simulink model "ILC_pidQuadsim"  (R2024b)
settings: Solver=VariableStepAuto  StartTime=0.0  StopTime=50  RelTol=1e-3
values from neighbouring files (symbols this model uses):
  tsamp_ILC = 0.10    (= 0.1)    [ILC_setup.m]
undefined symbols (not defined in the file or in its folder): A, B, C, D, pwm, quad
libraries: simulink x2, slctrlobsolete x2, realtime_pacer_lib x2
(part 1 of 2)
settings Model: Creator=elprof  LastModifiedBy=elprof

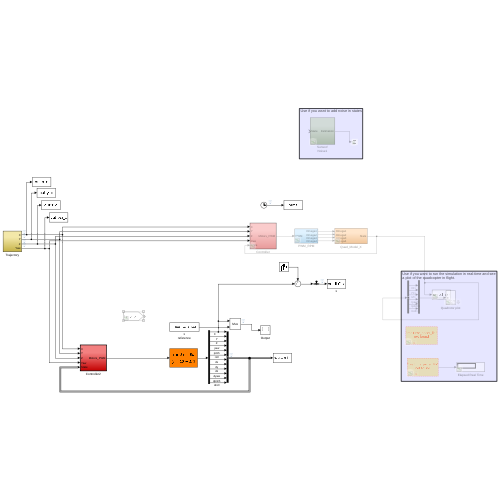
[thumbnail: Simulink's stored preview of the top-level diagram]
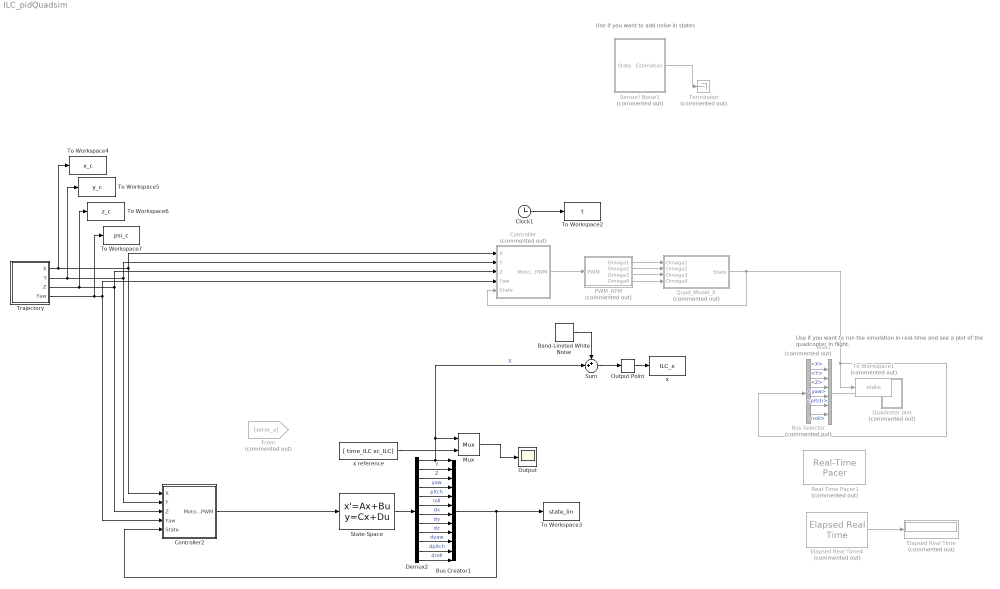
== system ILC_pidQuadsim ==
  note: Use if you want to add noise in states
  note: Use if you want to run the simulation in real-time and see
      | a plot of the quadcopter in flight.
  Band-Limited White Noise : simulink/Sources/Band-Limited White Noise  Cov=[0.0001]*0  Ts=0.1  seed=[23341]
  Bus Creator1 : BusCreator  Inputs=12
  Bus Selector : BusSelector  Commented=on  OutputSignals=X,Y,Z,yaw,pitch,roll
  Clock1 : Clock
  Controller : Subsystem  Commented=on  TreatAsAtomicUnit=on
  Controller2 : Subsystem  TreatAsAtomicUnit=on
  Demux2 : Demux  Outputs=12
  Elapsed Real Time : Display  Commented=on
      settings: Decimation=2
  Elapsed Real Time4 : realtime_pacer_lib/Elapsed Real Time  Commented=on
  From : From  Commented=on  GotoTag=error_x
  Mux : Mux  Inputs=2
  Mux1 : Mux  Commented=on  Inputs=6
  Output : Scope
  Output Point : slctrlobsolete/Output Point
  PWM_RPM : Subsystem  Commented=on
  Quad_Model_X : Subsystem  Commented=on
  Quadrotor plot : Subsystem  Commented=on  AncestorBlock=roblocks/Robot Graphics/Quadrotor plot  mask{quad=quad, xydim=2, zdim=2.3}
      mask prompts: quad "Model"; xydim "xy-axes dimension"; zdim "z-axis dimension"
      mask help: Animate quadrotor.
      mask Help:
      | This block graphically displays a quadrotor (flying robot).
      | 
      | A new figure is created and A graphical model of a quadrotor is animated
      | to a pose specified by the state vector input to the block.
      | 
      | The state vector is [x y z roll pitch yaw] in world coordinates and the
      | angles are in radians.
      | 
      | Notes:
      | - The dimensions of the vehicle workspace are set by parameters
  Real-Time Pacer1 : realtime_pacer_lib/Real-Time Pacer  Commented=on  simTimePerRealTime=1
  Sensor/ Noise1 : Subsystem  Commented=on
  State-Space : StateSpace  A=A  B=B  C=C  D=D  InitialCondition=[0 0 0 0 0 0 0 0 0 0 0 0]'
  Sum : Sum  Inputs=++|  InputSameDT=on  SaturateOnIntegerOverflow=on  OutDataTypeStr=Inherit: Same as first input
  Terminator : Terminator  Commented=on
  To Workspace1 : ToWorkspace  Commented=on  VariableName=state  SampleTime=-1
  To Workspace2 : ToWorkspace  VariableName=t  SampleTime=-1
  To Workspace3 : ToWorkspace  VariableName=state_lin  SampleTime=-1
  To Workspace4 : ToWorkspace  VariableName=x_c  SampleTime=-1
  To Workspace5 : ToWorkspace  VariableName=y_c  SampleTime=-1
  To Workspace6 : ToWorkspace  VariableName=z_c  SampleTime=-1
  To Workspace7 : ToWorkspace  VariableName=psi_c  SampleTime=-1
  Trajectory : Subsystem
  x : ToWorkspace  VariableName=ILC_x  SaveFormat=Structure With Time  SampleTime=-1
  x reference : FromWorkspace  VariableName=[ time_ILC xc_ILC]  SampleTime=tsamp_ILC  ZeroCross=off
  wires:
  Bus Selector/2 -> Mux1/2  "<Y>"
  PWM_RPM/3(Omega3) -> Quad_Model_X/3(Omega3)
  Bus Selector/4 -> Mux1/4  "<yaw>"
  PWM_RPM/2(Omega2) -> Quad_Model_X/2(Omega2)
  Demux2/10 -> Bus Creator1/10  "dyaw"
  PWM_RPM/1(Omega1) -> Quad_Model_X/1(Omega1)
  Demux2/8 -> Bus Creator1/8  "dy"
  Trajectory/2(Y) -> To Workspace5/1, Controller2/2(Y), Controller/2(Y)
  Controller2/1(Motors_PWM) -> State-Space/1
  Bus Selector/1 -> Mux1/1  "<X>"
  Bus Creator1/1 -> To Workspace3/1, Controller2/5(State)
  PWM_RPM/4(Omega4) -> Quad_Model_X/4(Omega4)
  Demux2/5 -> Bus Creator1/5  "pitch"
  Trajectory/3(Z) -> To Workspace6/1, Controller2/3(Z), Controller/3(Z)
  State-Space/1 -> Demux2/1
  Bus Selector/6 -> Mux1/6  "<roll>"
  Demux2/12 -> Bus Creator1/12  "droll"
  Mux1/1 -> Quadrotor plot/1(X)
  Demux2/6 -> Bus Creator1/6  "roll"
  Demux2/3 -> Bus Creator1/3  "Z"
  Demux2/9 -> Bus Creator1/9  "dz"
  Demux2/1 -> Sum/2, Mux/1, Bus Creator1/1  "X"
  Quad_Model_X/1(State) -> Controller/5(State), To Workspace1/1, Bus Selector/1
  Sensor/ Noise1/1(Estimation) -> Terminator/1
  Demux2/11 -> Bus Creator1/11  "dpitch"
  Controller/1(Motors_PWM) -> PWM_RPM/1(PWM)
  Demux2/2 -> Bus Creator1/2  "Y"
  Trajectory/4(Yaw) -> To Workspace7/1, Controller2/4(Yaw), Controller/4(Yaw)
  Demux2/7 -> Bus Creator1/7  "dx"
  Trajectory/1(X) -> To Workspace4/1, Controller2/1(X), Controller/1(X)
  Bus Selector/5 -> Mux1/5  "<pitch>"
  Elapsed Real Time4/1 -> Elapsed Real Time/1
  Clock1/1 -> To Workspace2/1
  Demux2/4 -> Bus Creator1/4  "yaw"
  Bus Selector/3 -> Mux1/3  "<Z>"
  x reference/1 -> Mux/2
  Output Point/1 -> x/1
  Mux/1 -> Output/1
  Sum/1 -> Output Point/1
  Band-Limited White Noise/1 -> Sum/1

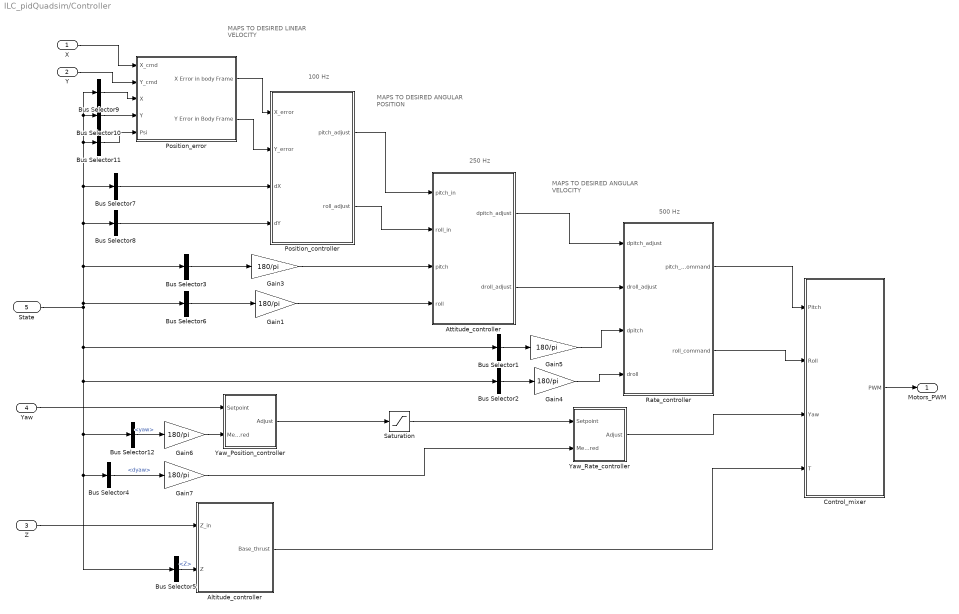
== system ILC_pidQuadsim/Controller ==
  note: 100 Hz
  note: MAPS TO DESIRED
      | ANGULAR VELOCITY
  note: MAPS TO DESIRED
      | ANGULAR POSITION
  note: MAPS TO DESIRED
      | LINEAR VELOCITY
  note: 250 Hz
  note: 500 Hz
  X : Inport
  Y : Inport  Port=2
  Z : Inport  Port=3
  Yaw : Inport  Port=4
  State : Inport  Port=5
  Altitude_controller : Subsystem
  Attitude_controller : Subsystem
  Bus Selector1 : BusSelector  OutputSignals=dpitch  OutputAsBus=on
  Bus Selector10 : BusSelector  OutputSignals=Y  OutputAsBus=on
  Bus Selector11 : BusSelector  OutputSignals=yaw  OutputAsBus=on
  Bus Selector12 : BusSelector  OutputSignals=yaw
  Bus Selector2 : BusSelector  OutputSignals=droll  OutputAsBus=on
  Bus Selector3 : BusSelector  OutputSignals=pitch  OutputAsBus=on
  Bus Selector4 : BusSelector  OutputSignals=dyaw
  Bus Selector5 : BusSelector  OutputSignals=Z
  Bus Selector6 : BusSelector  OutputSignals=roll  OutputAsBus=on
  Bus Selector7 : BusSelector  OutputSignals=dx  OutputAsBus=on
  Bus Selector8 : BusSelector  OutputSignals=dy  OutputAsBus=on
  Bus Selector9 : BusSelector  OutputSignals=X  OutputAsBus=on
  Control_mixer : Subsystem
  Gain{1,3..7} (6 alike) : Gain  Gain=180/pi
  Position_controller : Subsystem
  Position_error : Subsystem
  Rate_controller : Subsystem
  Saturation : Saturate  UpperLimit=200  LowerLimit=-200
  Yaw_Position_controller : Subsystem
  Yaw_Rate_controller : Subsystem
  Motors_PWM : Outport
  wires:
  Control_mixer/1(PWM) -> Motors_PWM/1
  Rate_controller/1(pitch_command) -> Control_mixer/1(Pitch)
  Rate_controller/2(roll_command) -> Control_mixer/2("Roll\t")
  Altitude_controller/1(Base_thrust) -> Control_mixer/4(T)
  Z/1 -> Altitude_controller/1(Z_in)
  Bus Selector5/1 -> Altitude_controller/2(Z)  "<Z>"
  Bus Selector4/1 -> Gain7/1  "<dyaw>"
  State/1 -> Bus Selector9/1, Bus Selector10/1, Bus Selector11/1, Bus Selector7/1, Bus Selector8/1, Bus Selector3/1, Bus Selector6/1, Bus Selector5/1, Bus Selector4/1, Bus Selector12/1, Bus Selector2/1, Bus Selector1/1
  Yaw_Position_controller/1(Adjust) -> Saturation/1
  Yaw_Rate_controller/1(Adjust) -> Control_mixer/3(Yaw)
  Bus Selector6/1 -> Gain1/1
  Attitude_controller/1(dpitch_adjust) -> Rate_controller/1(dpitch_adjust)
  Attitude_controller/2(droll_adjust) -> Rate_controller/2(droll_adjust)
  Bus Selector9/1 -> Position_error/3(X)
  Bus Selector10/1 -> Position_error/4(Y)
  Bus Selector11/1 -> Position_error/5(Psi)
  Position_error/1(X Error in body Frame) -> Position_controller/1(X_error)
  Position_error/2(Y Error in Body Frame) -> Position_controller/2(Y_error)
  Position_controller/1(pitch_adjust) -> Attitude_controller/1(pitch_in)
  Bus Selector3/1 -> Gain3/1
  Gain1/1 -> Attitude_controller/4(roll)
  Gain3/1 -> Attitude_controller/3(pitch)
  Gain4/1 -> Rate_controller/4(droll)
  Gain5/1 -> Rate_controller/3(dpitch)
  Bus Selector1/1 -> Gain5/1
  Bus Selector2/1 -> Gain4/1
  Bus Selector12/1 -> Gain6/1  "<yaw>"
  Gain6/1 -> Yaw_Position_controller/2(Measured)
  Gain7/1 -> Yaw_Rate_controller/2(Measured)
  Position_controller/2(roll_adjust) -> Attitude_controller/2(roll_in)
  X/1 -> Position_error/1(X_cmd)
  Y/1 -> Position_error/2(Y_cmd)
  Bus Selector7/1 -> Position_controller/3(dX)
  Bus Selector8/1 -> Position_controller/4(dY)
  Yaw/1 -> Yaw_Position_controller/1(Setpoint)
  Saturation/1 -> Yaw_Rate_controller/1(Setpoint)

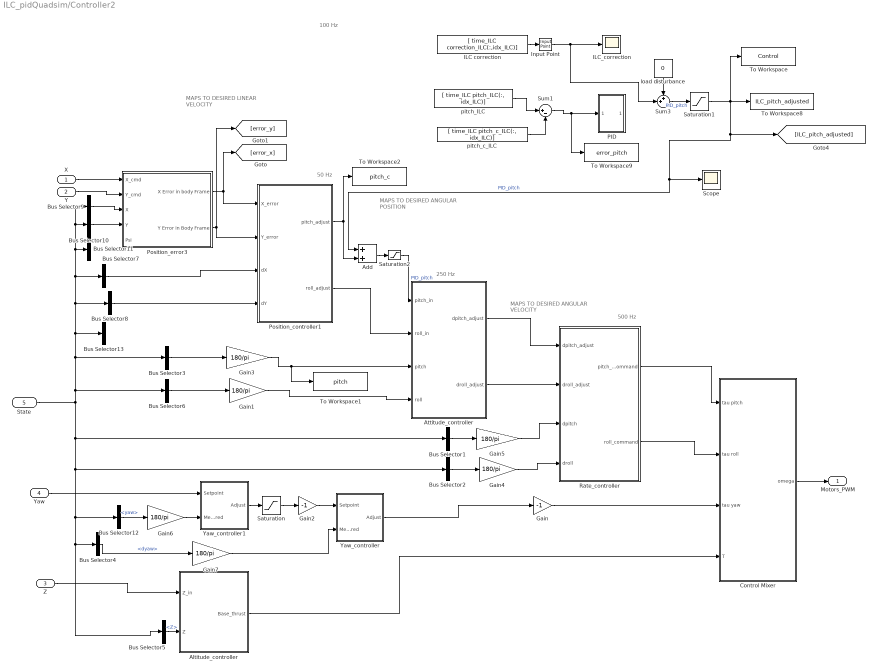
== system ILC_pidQuadsim/Controller2 ==
  note: 500 Hz
  note: 250 Hz
  note: 100 Hz
  note: MAPS TO DESIRED
      | LINEAR VELOCITY
  note: MAPS TO DESIRED
      | ANGULAR POSITION
  note: MAPS TO DESIRED
      | ANGULAR VELOCITY
  note: 50 Hz
  X : Inport
  Y : Inport  Port=2
  Z : Inport  Port=3
  Yaw : Inport  Port=4
  State : Inport  Port=5
  Add : Sum
  Altitude_controller : Subsystem
  Attitude_controller : Subsystem
  Bus Selector1 : BusSelector  OutputSignals=dpitch  OutputAsBus=on
  Bus Selector10 : BusSelector  OutputSignals=Y  OutputAsBus=on
  Bus Selector11 : BusSelector  OutputSignals=yaw  OutputAsBus=on
  Bus Selector12 : BusSelector  OutputSignals=yaw
  Bus Selector13 : BusSelector  OutputSignals=yaw  OutputAsBus=on
  Bus Selector2 : BusSelector  OutputSignals=droll  OutputAsBus=on
  Bus Selector3 : BusSelector  OutputSignals=pitch  OutputAsBus=on
  Bus Selector4 : BusSelector  OutputSignals=dyaw
  Bus Selector5 : BusSelector  OutputSignals=Z
  Bus Selector6 : BusSelector  OutputSignals=roll  OutputAsBus=on
  Bus Selector7 : BusSelector  OutputSignals=dx  OutputAsBus=on
  Bus Selector8 : BusSelector  OutputSignals=dy  OutputAsBus=on
  Bus Selector9 : BusSelector  OutputSignals=X  OutputAsBus=on
  Control Mixer : Subsystem  AncestorBlock=roblocks/Dynamics/Control Mixer 4
      mask help: Quadrotor control mixer
      mask Help:
      | Determine rotor speeds based on desired torques and thrust.
      | 
      | <b>Inputs::</b>
      | 
      | tau pitch (1x1)  desired pitching torque [Nm]
      | tau roll (1x1)   desired rolling torque [Nm]
      | tau yaw (1x1)    desired yawing torque [Nm]
      | T (1x1)          desired thrust [N]
      | 
      | <b>Outputs::</b>
      | 
      | w1 (1x1) angular velocity of rotor 1 [rad]
      | w2 (1x1) angular velocity of rotor 2 [rad]
      | w3 (1x1) angular velocity of rotor 3 [rad]
      | w4 (1x1) angular velocity of rotor 4 [rad]
      | 
      | <b>Notes::</b>
      | 
      | - Assumes the rotor labelling convention of RVC Fig 4.16.
      | - The quadrotor is underactuated and has only 4 inputs.
  Gain : Gain  Gain=-1
  Gain{1,3..7} (6 alike) : Gain  Gain=180/pi
  Gain2 : Gain  Gain=-1
  ILC correction : FromWorkspace  VariableName=[ time_ILC correction_ILC(:,idx_ILC)]  SampleTime=tsamp_ILC  ZeroCross=off
  ILC_correction : Scope
  Input Point : slctrlobsolete/Input Point
  PID : Subsystem  mask{K=0, Ti=100, Td=20}
  Position_controller1 : Subsystem
  Position_error3 : Subsystem
  Rate_controller : Subsystem
  Saturation : Saturate  UpperLimit=200  LowerLimit=-200
  Saturation1 : Saturate  UpperLimit=30  LowerLimit=-30
  Saturation2 : Saturate  UpperLimit=30  LowerLimit=-30
  Scope : Scope
  Sum1 : Sum  Inputs=|+-
  Sum3 : Sum  Inputs=++|  InputSameDT=on  SaturateOnIntegerOverflow=on  OutDataTypeStr=Inherit: Same as first input
  To Workspace : ToWorkspace  VariableName=Control  SaveFormat=Timeseries  SampleTime=-1
  To Workspace1 : ToWorkspace  VariableName=pitch  SaveFormat=Timeseries  SampleTime=-1
  To Workspace2 : ToWorkspace  VariableName=pitch_c  SampleTime=-1
  To Workspace8 : ToWorkspace  VariableName=ILC_pitch_adjusted  SaveFormat=Timeseries  SampleTime=-1
  To Workspace9 : ToWorkspace  VariableName=error_pitch  SaveFormat=Timeseries  SampleTime=-1
  Yaw_controller : Subsystem
  Yaw_controller1 : Subsystem
  load disturbance : Constant  Value=0
  pitch_ILC : FromWorkspace  VariableName=[ time_ILC pitch_ILC(:, idx_ILC)]  SampleTime=tsamp_ILC  ZeroCross=off
  pitch_c_ILC : FromWorkspace  VariableName="[ time_ILC  pitch_c_ILC(:, idx_ILC)]"  SampleTime=tsamp_ILC  ZeroCross=off
  Motors_PWM : Outport
  wires:
  Y/1 -> Position_error3/2(Y_cmd)
  X/1 -> Position_error3/1(X_cmd)
  Gain7/1 -> Yaw_controller/2(Measured)
  Gain6/1 -> Yaw_controller1/2(Measured)
  Bus Selector12/1 -> Gain6/1  "<yaw>"
  Bus Selector2/1 -> Gain4/1
  Bus Selector1/1 -> Gain5/1
  Gain5/1 -> Rate_controller/3(dpitch)
  Gain4/1 -> Rate_controller/4(droll)
  Gain3/1 -> To Workspace1/1, Attitude_controller/3(pitch)
  Gain1/1 -> Attitude_controller/4(roll)
  Bus Selector3/1 -> Gain3/1
  Position_controller1/1(pitch_adjust) -> Add/2, To Workspace2/1
  Bus Selector8/1 -> Position_controller1/4(dY)
  Bus Selector7/1 -> Position_controller1/3(dX)
  Position_error3/2(Y Error in Body Frame) -> Position_controller1/2(Y_error), [error_y]
  Position_error3/1(X Error in body Frame) -> Position_controller1/1(X_error), [error_x]
  Bus Selector10/1 -> Position_error3/4(Y)
  Bus Selector9/1 -> Position_error3/3(X)
  Attitude_controller/2(droll_adjust) -> Rate_controller/2(droll_adjust)
  Attitude_controller/1(dpitch_adjust) -> Rate_controller/1(dpitch_adjust)
  Bus Selector6/1 -> Gain1/1
  Saturation/1 -> Gain2/1
  Gain2/1 -> Yaw_controller/1(Setpoint)
  Yaw/1 -> Yaw_controller1/1(Setpoint)
  Yaw_controller/1(Adjust) -> Gain/1
  Gain/1 -> Control Mixer/3(tau yaw)
  Yaw_controller1/1(Adjust) -> Saturation/1
  State/1 -> Bus Selector1/1, Bus Selector2/1, Bus Selector12/1, Bus Selector4/1, Bus Selector5/1, Bus Selector3/1, Bus Selector7/1, Bus Selector10/1, Bus Selector9/1, Bus Selector11/1, Bus Selector8/1, Bus Selector13/1, Bus Selector6/1
  Bus Selector4/1 -> Gain7/1  "<dyaw>"
  Bus Selector5/1 -> Altitude_controller/2(Z)  "<Z>"
  Z/1 -> Altitude_controller/1(Z_in)
  Altitude_controller/1(Base_thrust) -> Control Mixer/4(T)
  Rate_controller/2(roll_command) -> Control Mixer/2(tau roll)
  Rate_controller/1(pitch_command) -> Control Mixer/1(tau pitch)
  Control Mixer/1(omega) -> Motors_PWM/1
  pitch_c_ILC/1 -> Sum1/2
  ILC correction/1 -> Input Point/1
  Input Point/1 -> Sum3/2, ILC_correction/1
  Sum1/1 -> To Workspace9/1, PID/1(In1)
  pitch_ILC/1 -> Sum1/1
  load disturbance/1 -> Sum3/1
  Sum3/1 -> Saturation1/1  "PID_pitch"
  Add/1 -> Saturation2/1
  Saturation2/1 -> Attitude_controller/1(pitch_in)  "PID_pitch"
  Saturation1/1 -> To Workspace/1, [ILC_pitch_adjusted], Add/1, Scope/1, To Workspace8/1  "PID_pitch"
  Position_controller1/2(roll_adjust) -> Attitude_controller/2(roll_in)

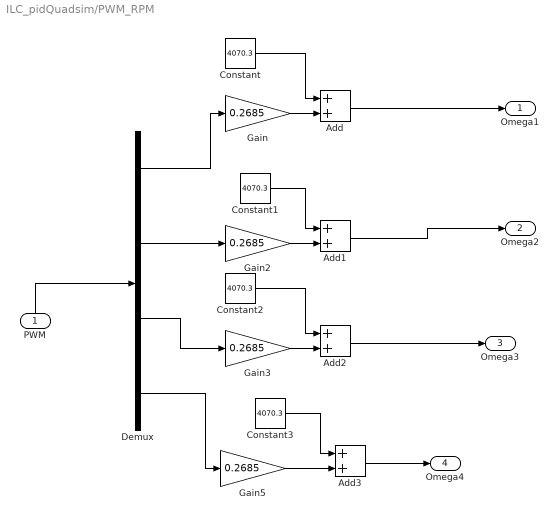
== system ILC_pidQuadsim/PWM_RPM ==
  PWM : Inport
  Add{,1..3} (4 alike) : Sum
  Constant{,1..3} (4 alike) : Constant  Value=4070.3
  Demux : Demux
  Gain{,2..3,5} (4 alike) : Gain  Gain=0.2685
  Omega1 : Outport
  Omega2 : Outport  Port=2
  Omega3 : Outport  Port=3
  Omega4 : Outport  Port=4
  wires:
  Gain/1 -> Add/2
  Demux/1 -> Gain/1
  Demux/4 -> Gain5/1
  Gain5/1 -> Add3/2
  Constant3/1 -> Add3/1
  Add3/1 -> Omega4/1
  Constant1/1 -> Add1/1
  Gain2/1 -> Add1/2
  Demux/2 -> Gain2/1
  Add1/1 -> Omega2/1
  PWM/1 -> Demux/1
  Add/1 -> Omega1/1
  Add2/1 -> Omega3/1
  Demux/3 -> Gain3/1
  Constant2/1 -> Add2/1
  Gain3/1 -> Add2/2
  Constant/1 -> Add/1

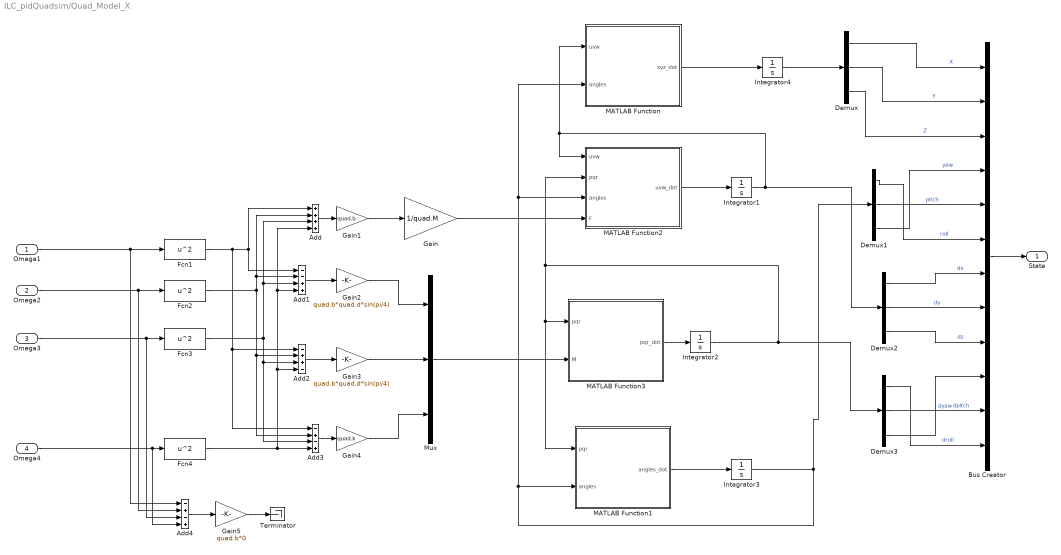
== system ILC_pidQuadsim/Quad_Model_X ==
  Omega1 : Inport
  Omega2 : Inport  Port=2
  Omega3 : Inport  Port=3
  Omega4 : Inport  Port=4
  Add : Sum  Inputs=++++
  Add1 : Sum  Inputs=--++
  Add2 : Sum  Inputs=-++-
  Add3 : Sum  Inputs=-+-+
  Add4 : Sum  Inputs=-+-+
  Bus Creator : BusCreator  Inputs=12
  Demux{,1..3} (4 alike) : Demux  Outputs=3
  Fcn{1..4} (4 alike) : Fcn  Expr=u^2
  Gain : Gain  Gain=1/quad.M
  Gain1 : Gain  Gain=quad.b
  Gain2 : Gain  Gain=quad.b*quad.d*sin(pi/4)
  Gain3 : Gain  Gain=quad.b*quad.d*sin(pi/4)
  Gain4 : Gain  Gain=quad.k
  Gain5 : Gain  Gain=quad.b*0
  Integrator1 : Integrator
  Integrator2 : Integrator
  Integrator3 : Integrator
  Integrator4 : Integrator  InitialCondition=[0;0;0]
  MATLAB Function : MATLAB Function  TreatAsAtomicUnit=on
  MATLAB Function1 : MATLAB Function  TreatAsAtomicUnit=on
  MATLAB Function2 : MATLAB Function  TreatAsAtomicUnit=on
  MATLAB Function3 : MATLAB Function  TreatAsAtomicUnit=on
  Mux : Mux  Inputs=3
  Terminator : Terminator
  State : Outport
  wires:
  Gain1/1 -> Gain/1
  Fcn4/1 -> Add/4, Add1/4, Add2/4, Add3/4
  Fcn3/1 -> Add1/3, Add/3, Add2/3, Add3/3
  Fcn2/1 -> Add2/2, Add3/2, Add1/2, Add/2
  Fcn1/1 -> Add/1, Add1/1, Add2/1, Add3/1
  Bus Creator/1 -> State/1
  Add1/1 -> Gain2/1
  Add/1 -> Gain1/1
  Omega2/1 -> Add4/2, Fcn2/1
  Omega1/1 -> Fcn1/1, Add4/1
  Add2/1 -> Gain3/1
  Gain2/1 -> Mux/1
  Gain4/1 -> Mux/3
  Omega3/1 -> Add4/3, Fcn3/1
  Omega4/1 -> Fcn4/1, Add4/4
  Add4/1 -> Gain5/1
  Add3/1 -> Gain4/1
  Gain3/1 -> Mux/2
  Gain/1 -> MATLAB Function2/4(F)
  Mux/1 -> MATLAB Function3/2(M)
  MATLAB Function/1(xyz_dot) -> Integrator4/1
  MATLAB Function2/1(uvw_dot) -> Integrator1/1
  MATLAB Function3/1(pqr_dot) -> Integrator2/1
  MATLAB Function1/1(angles_dot) -> Integrator3/1
  Integrator3/1 -> Demux1/1, MATLAB Function/2(angles), MATLAB Function2/3(angles), MATLAB Function1/2(angles)
  Integrator1/1 -> Demux2/1, MATLAB Function/1(uvw), MATLAB Function2/1(uvw)
  Integrator2/1 -> Demux3/1, MATLAB Function2/2(pqr), MATLAB Function1/1(pqr), MATLAB Function3/1(pqr)
  Integrator4/1 -> Demux/1
  Demux/1 -> Bus Creator/1  "X"
  Demux/2 -> Bus Creator/2  "Y"
  Demux/3 -> Bus Creator/3  "Z"
  Demux1/3 -> Bus Creator/4  "yaw"
  Demux1/1 -> Bus Creator/6  "roll"
  Demux2/1 -> Bus Creator/7  "dx"
  Demux2/2 -> Bus Creator/8  "dy"
  Demux2/3 -> Bus Creator/9  "dz"
  Demux3/3 -> Bus Creator/10  "dyaw"
  Demux3/2 -> Bus Creator/11  "dpitch"
  Demux3/1 -> Bus Creator/12  "droll"
  Gain5/1 -> Terminator/1
  Demux1/2 -> Bus Creator/5  "pitch"

== system ILC_pidQuadsim/Quadrotor plot ==
  X : Inport
  Plotter : S-Function  FunctionName=quadrotor_plot  Parameters=[xydim, zdim], 1, 1,quad  SFunctionDeploymentMode=off  EnableBusSupport=off
  wires:
  X/1 -> Plotter/1

== system ILC_pidQuadsim/Sensor// Noise1 ==
  note: state
  State : Inport
  Bus Creator : BusCreator  Inputs=2
  Bus Creator1 : BusCreator  Inputs=3
  Bus Selector7 : BusSelector  OutputSignals=X,Y,Z
  Bus Selector8 : BusSelector  OutputSignals=yaw,pitch,roll,dx,dy,dz,dyaw,dpitch,droll  OutputAsBus=on
  Error_X1 : Gain  Gain=0.04
  Error_Y : Gain  Gain=0.04
  Error_Z : Gain  Gain=0.04
  Random Number1 : RandomNumber  SampleTime=0.1
  Random Number2 : RandomNumber  SampleTime=0.1
  Random Number3 : RandomNumber  SampleTime=0.1
  Sum5 : Sum  Inputs=++|
  Sum6 : Sum  Inputs=++|
  Sum7 : Sum  Inputs=++|
  Estimation : Outport
  wires:
  State/1 -> Bus Selector8/1, Bus Selector7/1
  Error_X1/1 -> Sum5/1
  Bus Selector8/1 -> Bus Creator/2
  Random Number3/1 -> Error_X1/1
  Bus Creator/1 -> Estimation/1
  Bus Selector7/1 -> Sum5/2  "<X>"
  Bus Selector7/2 -> Sum6/2  "<Y>"
  Bus Selector7/3 -> Sum7/2  "<Z>"
  Sum5/1 -> Bus Creator1/1  "X'"
  Sum6/1 -> Bus Creator1/2  "Y'"
  Sum7/1 -> Bus Creator1/3  "Z'"
  Bus Creator1/1 -> Bus Creator/1
  Random Number1/1 -> Error_Y/1
  Error_Y/1 -> Sum6/1
  Random Number2/1 -> Error_Z/1
  Error_Z/1 -> Sum7/1

== system ILC_pidQuadsim/Trajectory ==
  Constant3 : Constant
  Ramp2 : simulink/Sources/Ramp  slope=60  start=0  InitialOutput=0
  x* : Sin  Amplitude=0.8  Frequency=2*pi*0.085  Phase=0-0.1  SampleTime=0
  y*1 : Sin  Amplitude=0.8  Frequency=2*pi*0.085  Phase=pi/2-0.1  SampleTime=0
  X : Outport
  Y : Outport  Port=2
  Z : Outport  Port=3
  Yaw : Outport  Port=4
  wires:
  Ramp2/1 -> Yaw/1
  y*1/1 -> Y/1
  x*/1 -> X/1
  Constant3/1 -> Z/1

== system ILC_pidQuadsim/Controller/Altitude_controller ==
  Z_in : Inport
  Z : Inport  Port=2
  "Min_thrust " : Constant  Value=pwm  SampleTime=0
  PID_Altitude : Subsystem
  Saturation : Saturate  UpperLimit=60000  LowerLimit=-20000
  Saturation1 : Saturate  UpperLimit=15000  LowerLimit=-20000
  Sum3 : Sum  Inputs=|++
  Base_thrust : Outport
  wires:
  Saturation/1 -> Base_thrust/1
  "Min_thrust "/1 -> Sum3/2
  Sum3/1 -> Saturation/1
  Z/1 -> PID_Altitude/2(Measured)
  Z_in/1 -> PID_Altitude/1(Setpoint)
  Saturation1/1 -> Sum3/1
  PID_Altitude/1(Adjust) -> Saturation1/1

== system ILC_pidQuadsim/Controller/Attitude_controller ==
  pitch_in : Inport
  roll_in : Inport  Port=2
  pitch : Inport  Port=3
  roll : Inport  Port=4
  PID_Pitch1 : Subsystem
  PID_Pitch3 : Subsystem
  PID_Pitch_Rate2 : Subsystem
  PID_Roll_Rate1 : Subsystem
  dpitch_adjust : Outport
  droll_adjust : Outport  Port=2
  wires:
  roll_in/1 -> PID_Roll_Rate1/1(Setpoint)
  roll/1 -> PID_Roll_Rate1/2(Measured)
  PID_Roll_Rate1/1(Adjust) -> droll_adjust/1
  pitch_in/1 -> PID_Pitch_Rate2/1(Setpoint)
  pitch/1 -> PID_Pitch_Rate2/2(Measured)
  PID_Pitch_Rate2/1(Adjust) -> dpitch_adjust/1

== system ILC_pidQuadsim/Controller/Control_mixer ==
  Pitch : Inport
  "Roll\t" : Inport  Port=2
  Yaw : Inport  Port=3
  T : Inport  Port=4
  Configuration_+ : Subsystem
  Configuration_X1 : Subsystem
  Mode_Selector : Constant  Value=2
  Multiport Switch : MultiPortSwitch  Inputs=2  SaturateOnIntegerOverflow=off  InputSameDT=off
  Mux : Mux
  Mux1 : Mux
  PWM : Outport
  wires:
  Pitch/1 -> Configuration_X1/1(Pitch), Configuration_+/1(Pitch)
  Configuration_X1/3(W3) -> Mux1/3
  Mux1/1 -> Multiport Switch/3
  Mux/1 -> Multiport Switch/2
  Configuration_X1/4(W4) -> Mux1/4
  T/1 -> Configuration_X1/4(Tau), Configuration_+/4(Tau)
  Multiport Switch/1 -> PWM/1
  Yaw/1 -> Configuration_X1/3(Yaw), Configuration_+/3(Yaw)
  "Roll\t"/1 -> Configuration_X1/2(Roll), Configuration_+/2(Roll)
  Mode_Selector/1 -> Multiport Switch/1
  Configuration_+/2(W2) -> Mux/2
  Configuration_+/1(W1) -> Mux/1
  Configuration_X1/2(W2) -> Mux1/2
  Configuration_X1/1(W1) -> Mux1/1
  Configuration_+/3(W3) -> Mux/3
  Configuration_+/4(W4) -> Mux/4

== system ILC_pidQuadsim/Controller/Position_controller ==
  X_error : Inport
  Y_error : Inport  Port=2
  dX : Inport  Port=3
  dY : Inport  Port=4
  PID_Roll_Rate2 : Subsystem
  PID_Roll_Rate3 : Subsystem
  PID_X2 : Subsystem
  PID_Y2 : Subsystem
  Saturation : Saturate  UpperLimit=30  LowerLimit=-30
  Saturation1 : Saturate  UpperLimit=30  LowerLimit=-30
  Scope1 : Scope
  Scope2 : Scope
  pitch_adjust : Outport
  roll_adjust : Outport  Port=2
  wires:
  Saturation1/1 -> roll_adjust/1
  PID_Roll_Rate3/1(Adjust) -> Saturation1/1
  Saturation/1 -> pitch_adjust/1, Scope1/1
  PID_Roll_Rate2/1(Adjust) -> Saturation/1, Scope2/1
  dX/1 -> PID_Roll_Rate2/2(Measured)
  X_error/1 -> PID_Roll_Rate2/1(Setpoint)
  dY/1 -> PID_Roll_Rate3/2(Measured)
  Y_error/1 -> PID_Roll_Rate3/1(Setpoint)

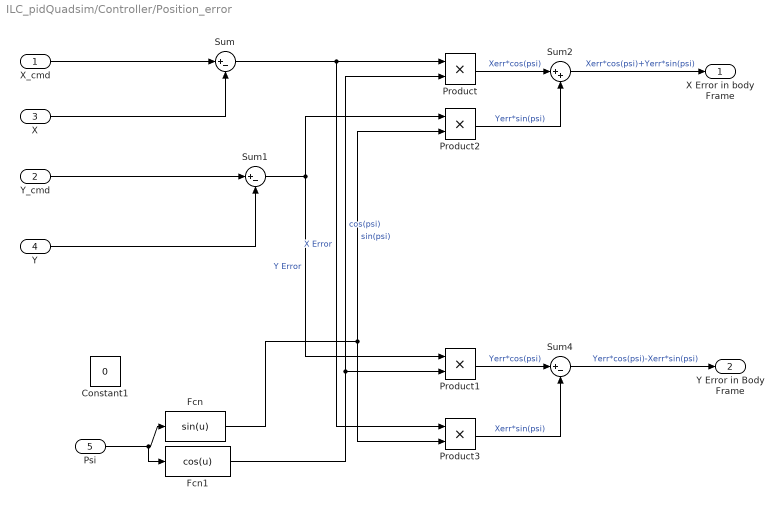
== system ILC_pidQuadsim/Controller/Position_error ==
  X_cmd : Inport
  Y_cmd : Inport  Port=2
  X : Inport  Port=3
  Y : Inport  Port=4
  Psi : Inport  Port=5
  Constant1 : Constant  Value=0
  Fcn : Fcn  Expr=sin(u)
  Fcn1 : Fcn  Expr=cos(u)
  Product{,1..3} (4 alike) : Product
  Sum : Sum  Inputs=|+-
  Sum1 : Sum  Inputs=|+-
  Sum2 : Sum  Inputs=|++
  Sum4 : Sum  Inputs=|+-
  X Error in body Frame : Outport
  Y Error in Body Frame : Outport  Port=2
  wires:
  Sum4/1 -> Y Error in Body Frame/1  "Yerr*cos(psi)-Xerr*sin(psi)"
  Product3/1 -> Sum4/2  "Xerr*sin(psi)"
  Sum1/1 -> Product2/1, Product1/1  "Y Error"
  Fcn/1 -> Product3/2, Product2/2  "sin(psi)"
  Sum2/1 -> X Error in body Frame/1  "Xerr*cos(psi)+Yerr*sin(psi)"
  Y_cmd/1 -> Sum1/1
  X_cmd/1 -> Sum/1
  X/1 -> Sum/2
  Y/1 -> Sum1/2
  Sum/1 -> Product3/1, Product/1  "X Error"
  Fcn1/1 -> Product/2, Product1/2  "cos(psi)"
  Product/1 -> Sum2/1  "Xerr*cos(psi)"
  Product2/1 -> Sum2/2  "Yerr*sin(psi)"
  Product1/1 -> Sum4/1  "Yerr*cos(psi)"
  Psi/1 -> Fcn1/1, Fcn/1

== system ILC_pidQuadsim/Controller/Rate_controller ==
  dpitch_adjust : Inport
  droll_adjust : Inport  Port=2
  dpitch : Inport  Port=3
  droll : Inport  Port=4
  PID_Pitch_Rate1 : Subsystem
  PID_Pitch_Rate3 : Subsystem
  PID_Roll_Rate1 : Subsystem
  PID_Roll_Rate3 : Subsystem
  pitch_command : Outport
  roll_command : Outport  Port=2
  wires:
  dpitch_adjust/1 -> PID_Roll_Rate3/1(Setpoint)
  PID_Roll_Rate3/1(Adjust) -> pitch_command/1
  droll_adjust/1 -> PID_Roll_Rate1/1(Setpoint)
  droll/1 -> PID_Roll_Rate1/2(Measured)
  PID_Roll_Rate1/1(Adjust) -> roll_command/1
  dpitch/1 -> PID_Roll_Rate3/2(Measured)

== system ILC_pidQuadsim/Controller/Yaw_Position_controller ==
  Setpoint : Inport
  Measured : Inport  Port=2
  1/dt : Gain  Gain=1/100  OutMin=[-200]  OutMax=[200]
  Kd : Gain  Gain=0  OutMin=[-200]  OutMax=[200]
  Ki : Gain  Gain=0  OutMin=[-200]  OutMax=[200]
  Kp : Gain  Gain=3  OutMin=[-200]  OutMax=[200]
  Memory : Memory
  Memory1 : Memory
  Saturation : Saturate  UpperLimit=166.7  LowerLimit=-166.7
  Sum1 : Sum  Inputs=|++
  Sum2 : Sum  Inputs=|+-
  Sum5 : Sum  Inputs=+++
  Sum6 : Sum  Inputs=+-|
  dt : Gain  Gain=1/100  OutMin=[-200]  OutMax=[200]
  Adjust : Outport
  wires:
  Measured/1 -> Sum6/2  "measured"
  Setpoint/1 -> Sum6/1  "pid_desired"
  Memory/1 -> Sum2/2  "pid_prevError"
  Ki/1 -> Sum5/2
  Sum5/1 -> Adjust/1
  Kp/1 -> Sum5/1
  Kd/1 -> Sum5/3
  dt/1 -> Sum1/1
  Sum2/1 -> 1/dt/1
  1/dt/1 -> Kd/1
  Sum6/1 -> Sum2/1, Memory/1, dt/1, Kp/1  "pid_error"
  Sum1/1 -> Memory1/1, Saturation/1  "pid_integ"
  Memory1/1 -> Sum1/2
  Saturation/1 -> Ki/1

== system ILC_pidQuadsim/Controller/Yaw_Rate_controller ==
  Setpoint : Inport
  Measured : Inport  Port=2
  1/dt : Gain  Gain=1/500  OutMin=[-200]  OutMax=[200]
  Kd : Gain  Gain=0  OutMin=[-200]  OutMax=[200]
  Ki : Gain  Gain=16.7  OutMin=[-200]  OutMax=[200]
  Kp : Gain  Gain=70  OutMin=[-200]  OutMax=[200]
  Memory : Memory
  Memory1 : Memory
  Saturation : Saturate  UpperLimit=166.7  LowerLimit=-166.7
  Sum1 : Sum  Inputs=|++
  Sum2 : Sum  Inputs=|+-
  Sum5 : Sum  Inputs=+++
  Sum6 : Sum  Inputs=+-|
  dt : Gain  Gain=1/500  OutMin=[-200]  OutMax=[200]
  Adjust : Outport
  wires:
  Measured/1 -> Sum6/2  "measured"
  Setpoint/1 -> Sum6/1  "pid_desired"
  Memory/1 -> Sum2/2  "pid_prevError"
  Ki/1 -> Sum5/2
  Sum5/1 -> Adjust/1
  Kp/1 -> Sum5/1
  Kd/1 -> Sum5/3
  dt/1 -> Sum1/1
  Sum2/1 -> 1/dt/1
  1/dt/1 -> Kd/1
  Sum6/1 -> Sum2/1, Memory/1, dt/1, Kp/1  "pid_error"
  Sum1/1 -> Memory1/1, Saturation/1  "pid_integ"
  Memory1/1 -> Sum1/2
  Saturation/1 -> Ki/1

== system ILC_pidQuadsim/Controller2/Altitude_controller ==
  Z_in : Inport
  Z : Inport  Port=2
  "Min_thrust " : Constant  Value=0  SampleTime=0
  PID_Altitude : Subsystem
  Saturation : Saturate  UpperLimit=60000  LowerLimit=-20000
  Saturation1 : Saturate  UpperLimit=15000  LowerLimit=-20000
  Sum3 : Sum  Inputs=|++
  Base_thrust : Outport
  wires:
  PID_Altitude/1(Adjust) -> Saturation1/1
  Saturation1/1 -> Sum3/1
  Z_in/1 -> PID_Altitude/1(Setpoint)
  Z/1 -> PID_Altitude/2(Measured)
  Sum3/1 -> Saturation/1
  "Min_thrust "/1 -> Sum3/2
  Saturation/1 -> Base_thrust/1

== system ILC_pidQuadsim/Controller2/Attitude_controller ==
  pitch_in : Inport
  roll_in : Inport  Port=2
  pitch : Inport  Port=3
  roll : Inport  Port=4
  PID_Pitch1 : Subsystem
  PID_Pitch3 : Subsystem
  PID_Roll_Rate1 : Subsystem
  PID_Roll_Rate2 : Subsystem
  dpitch_adjust : Outport
  droll_adjust : Outport  Port=2
  wires:
  PID_Roll_Rate2/1(Adjust) -> dpitch_adjust/1
  pitch/1 -> PID_Roll_Rate2/2(Measured)
  pitch_in/1 -> PID_Roll_Rate2/1(Setpoint)
  PID_Roll_Rate1/1(Adjust) -> droll_adjust/1
  roll/1 -> PID_Roll_Rate1/2(Measured)
  roll_in/1 -> PID_Roll_Rate1/1(Setpoint)

== system ILC_pidQuadsim/Controller2/Control Mixer ==
  tau pitch : Inport
  tau roll : Inport  Port=2
  tau yaw : Inport  Port=3
  T : Inport  Port=4
  Configuration_+ : Subsystem
  Configuration_X1 : Subsystem
  Configuration_X2 : Subsystem
  Mode_Selector : Constant  Value=2
  Multiport Switch : MultiPortSwitch  Inputs=2  SaturateOnIntegerOverflow=off  InputSameDT=off
  Mux : Mux
  Mux1 : Mux
  omega : Outport
  wires:
  Mux/1 -> Multiport Switch/2
  Multiport Switch/1 -> omega/1
  Mode_Selector/1 -> Multiport Switch/1
  T/1 -> Configuration_+/4(Tau), Configuration_X1/4(Tau)
  tau yaw/1 -> Configuration_+/3(Yaw), Configuration_X1/3(Yaw)
  tau roll/1 -> Configuration_+/2(Roll), Configuration_X1/2(Roll)
  tau pitch/1 -> Configuration_+/1(Pitch), Configuration_X1/1(Pitch)
  Mux1/1 -> Multiport Switch/3
  Configuration_X1/4(W4) -> Mux1/4
  Configuration_X1/3(W3) -> Mux1/3
  Configuration_X1/2(W2) -> Mux1/2
  Configuration_X1/1(W1) -> Mux1/1
  Configuration_+/4(W4) -> Mux/4
  Configuration_+/3(W3) -> Mux/3
  Configuration_+/2(W2) -> Mux/2
  Configuration_+/1(W1) -> Mux/1

== system ILC_pidQuadsim/Controller2/PID ==
  In1 : Inport
  1/Ti : Gain  Gain=1/Ti  SaturateOnIntegerOverflow=on  OutDataTypeStr=Inherit: Same as input  ParamDataTypeStr=Inherit: Same as input
  Integrator : Integrator
  K : Gain  Gain=K  SaturateOnIntegerOverflow=on  OutDataTypeStr=Inherit: Same as input  ParamDataTypeStr=Inherit: Same as input
  Sum1 : Sum  Inputs=+++  InputSameDT=on  SaturateOnIntegerOverflow=on  OutDataTypeStr=Inherit: Same as first input
  Transfer Fcn1 : TransferFcn  Numerator=[Td 0]  Denominator=[Td/10 1]
  Out1 : Outport
  wires:
  In1/1 -> K/1
  K/1 -> 1/Ti/1, Transfer Fcn1/1, Sum1/1
  1/Ti/1 -> Integrator/1
  Sum1/1 -> Out1/1
  Integrator/1 -> Sum1/2
  Transfer Fcn1/1 -> Sum1/3

== system ILC_pidQuadsim/Controller2/Position_controller1 ==
  X_error : Inport
  Y_error : Inport  Port=2
  dX : Inport  Port=3
  dY : Inport  Port=4
  PID_Roll_Rate2 : Subsystem
  PID_Roll_Rate3 : Subsystem
  PID_X2 : Subsystem
  PID_Y2 : Subsystem
  Saturation : Saturate  UpperLimit=30  LowerLimit=-30
  Saturation1 : Saturate  UpperLimit=30  LowerLimit=-30
  Scope1 : Scope
  Scope2 : Scope
  pitch_adjust : Outport
  roll_adjust : Outport  Port=2
  wires:
  PID_Roll_Rate3/1(Adjust) -> Saturation1/1
  Y_error/1 -> PID_Roll_Rate3/1(Setpoint)
  Saturation1/1 -> roll_adjust/1
  dY/1 -> PID_Roll_Rate3/2(Measured)
  dX/1 -> PID_Roll_Rate2/2(Measured)
  Saturation/1 -> Scope1/1, pitch_adjust/1
  X_error/1 -> PID_Roll_Rate2/1(Setpoint)
  PID_Roll_Rate2/1(Adjust) -> Scope2/1, Saturation/1

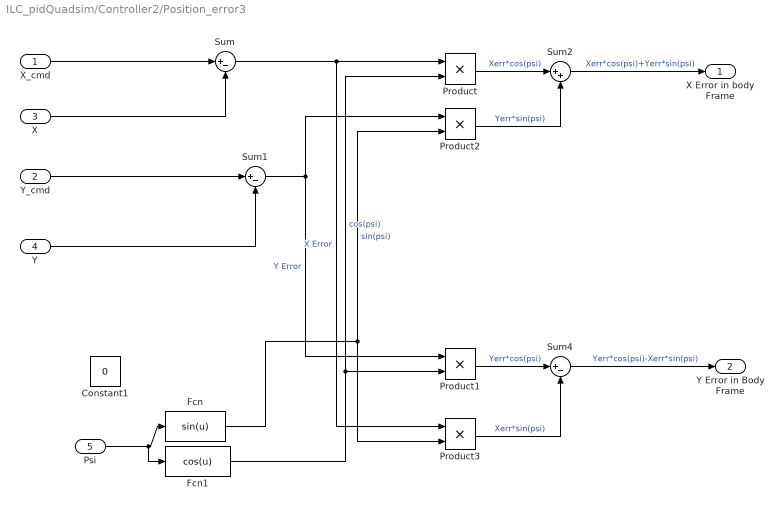
== system ILC_pidQuadsim/Controller2/Position_error3 ==
  X_cmd : Inport
  Y_cmd : Inport  Port=2
  X : Inport  Port=3
  Y : Inport  Port=4
  Psi : Inport  Port=5
  Constant1 : Constant  Value=0
  Fcn : Fcn  Expr=sin(u)
  Fcn1 : Fcn  Expr=cos(u)
  Product{,1..3} (4 alike) : Product
  Sum : Sum  Inputs=|+-
  Sum1 : Sum  Inputs=|+-
  Sum2 : Sum  Inputs=|++
  Sum4 : Sum  Inputs=|+-
  X Error in body Frame : Outport
  Y Error in Body Frame : Outport  Port=2
  wires:
  Psi/1 -> Fcn/1, Fcn1/1
  Product1/1 -> Sum4/1  "Yerr*cos(psi)"
  Product2/1 -> Sum2/2  "Yerr*sin(psi)"
  Product/1 -> Sum2/1  "Xerr*cos(psi)"
  Fcn1/1 -> Product1/2, Product/2  "cos(psi)"
  Sum/1 -> Product/1, Product3/1  "X Error"
  Y/1 -> Sum1/2
  X/1 -> Sum/2
  X_cmd/1 -> Sum/1
  Y_cmd/1 -> Sum1/1
  Sum2/1 -> X Error in body Frame/1  "Xerr*cos(psi)+Yerr*sin(psi)"
  Fcn/1 -> Product2/2, Product3/2  "sin(psi)"
  Sum1/1 -> Product1/1, Product2/1  "Y Error"
  Product3/1 -> Sum4/2  "Xerr*sin(psi)"
  Sum4/1 -> Y Error in Body Frame/1  "Yerr*cos(psi)-Xerr*sin(psi)"

== system ILC_pidQuadsim/Controller2/Rate_controller ==
  dpitch_adjust : Inport
  droll_adjust : Inport  Port=2
  dpitch : Inport  Port=3
  droll : Inport  Port=4
  PID_Pitch_Rate1 : Subsystem
  PID_Pitch_Rate3 : Subsystem
  PID_Roll_Rate1 : Subsystem
  PID_Roll_Rate3 : Subsystem
  pitch_command : Outport
  roll_command : Outport  Port=2
  wires:
  dpitch/1 -> PID_Roll_Rate3/2(Measured)
  PID_Roll_Rate1/1(Adjust) -> roll_command/1
  droll/1 -> PID_Roll_Rate1/2(Measured)
  droll_adjust/1 -> PID_Roll_Rate1/1(Setpoint)
  PID_Roll_Rate3/1(Adjust) -> pitch_command/1
  dpitch_adjust/1 -> PID_Roll_Rate3/1(Setpoint)

== system ILC_pidQuadsim/Controller2/Yaw_controller ==
  Setpoint : Inport
  Measured : Inport  Port=2
  1/dt : Gain  Gain=1/500  OutMin=[-200]  OutMax=[200]
  Kd : Gain  Gain=0  OutMin=[-200]  OutMax=[200]
  Ki : Gain  Gain=16.7  OutMin=[-200]  OutMax=[200]
  Kp : Gain  Gain=70  OutMin=[-200]  OutMax=[200]
  Memory : Memory
  Memory1 : Memory
  Saturation : Saturate  UpperLimit=166.7  LowerLimit=-166.7
  Sum1 : Sum  Inputs=|++
  Sum2 : Sum  Inputs=|+-
  Sum5 : Sum  Inputs=+++
  Sum6 : Sum  Inputs=+-|
  dt : Gain  Gain=1/500  OutMin=[-200]  OutMax=[200]
  Adjust : Outport
  wires:
  Saturation/1 -> Ki/1
  Memory1/1 -> Sum1/2
  Sum1/1 -> Saturation/1, Memory1/1  "pid_integ"
  Sum6/1 -> Kp/1, dt/1, Memory/1, Sum2/1  "pid_error"
  1/dt/1 -> Kd/1
  Sum2/1 -> 1/dt/1
  dt/1 -> Sum1/1
  Kd/1 -> Sum5/3
  Kp/1 -> Sum5/1
  Sum5/1 -> Adjust/1
  Ki/1 -> Sum5/2
  Memory/1 -> Sum2/2  "pid_prevError"
  Setpoint/1 -> Sum6/1  "pid_desired"
  Measured/1 -> Sum6/2  "measured"

== system ILC_pidQuadsim/Controller2/Yaw_controller1 ==
  Setpoint : Inport
  Measured : Inport  Port=2
  1/dt : Gain  Gain=1/100  OutMin=[-200]  OutMax=[200]
  Kd : Gain  Gain=0  OutMin=[-200]  OutMax=[200]
  Ki : Gain  Gain=0  OutMin=[-200]  OutMax=[200]
  Kp : Gain  Gain=-3  OutMin=[-200]  OutMax=[200]
  Memory : Memory
  Memory1 : Memory
  Saturation : Saturate  UpperLimit=166.7  LowerLimit=-166.7
  Sum1 : Sum  Inputs=|++
  Sum2 : Sum  Inputs=|+-
  Sum5 : Sum  Inputs=+++
  Sum6 : Sum  Inputs=+-|
  dt : Gain  Gain=1/100  OutMin=[-200]  OutMax=[200]
  Adjust : Outport
  wires:
  Saturation/1 -> Ki/1
  Memory1/1 -> Sum1/2
  Sum1/1 -> Saturation/1, Memory1/1  "pid_integ"
  Sum6/1 -> [error_yaw], Kp/1, dt/1, Memory/1, Sum2/1  "pid_error"
  1/dt/1 -> Kd/1
  Sum2/1 -> 1/dt/1
  dt/1 -> Sum1/1
  Kd/1 -> Sum5/3
  Kp/1 -> Sum5/1
  Sum5/1 -> Adjust/1
  Ki/1 -> Sum5/2
  Memory/1 -> Sum2/2  "pid_prevError"
  Setpoint/1 -> Sum6/1  "pid_desired"
  Measured/1 -> Sum6/2  "measured"

== system ILC_pidQuadsim/Controller/Altitude_controller/PID_Altitude ==
  Setpoint : Inport
  Measured : Inport  Port=2
  Derivative : Derivative
  Integrator Limited : Integrator  LimitOutput=on  UpperSaturationLimit=1000  LowerSaturationLimit=-1000
  Kd : Gain  Gain=9000  OutMin=[-200]  OutMax=[200]
  Ki : Gain  Gain=3500  OutMin=[-200]  OutMax=[200]
  Kp : Gain  Gain=11000  OutMin=[-200]  OutMax=[200]
  Sum5 : Sum  Inputs=+++
  Sum6 : Sum  Inputs=+-|
  Adjust : Outport
  wires:
  Derivative/1 -> Kd/1
  Integrator Limited/1 -> Ki/1
  Sum6/1 -> Kp/1, Integrator Limited/1, Derivative/1  "pid_error"
  Kd/1 -> Sum5/3
  Kp/1 -> Sum5/1
  Ki/1 -> Sum5/2
  Setpoint/1 -> Sum6/1  "pid_desired"
  Measured/1 -> Sum6/2  "measured"
  Sum5/1 -> Adjust/1

== system ILC_pidQuadsim/Controller/Attitude_controller/PID_Pitch1 ==
  Setpoint : Inport
  Measured : Inport  Port=2
  1/dt : Gain  Gain=250  OutMin=[-200]  OutMax=[200]
  Kd : Gain  Gain=0  OutMin=[-200]  OutMax=[200]
  Ki : Gain  Gain=0  OutMin=[-200]  OutMax=[200]
  Kp : Gain  Gain=3.5  OutMin=[-200]  OutMax=[200]
  Memory : Memory
  Memory1 : Memory
  Saturation : Saturate  UpperLimit=20  LowerLimit=-20
  Sum1 : Sum  Inputs=|++
  Sum2 : Sum  Inputs=|+-
  Sum5 : Sum  Inputs=+++
  Sum6 : Sum  Inputs=+-|
  dt : Gain  Gain=1/250  OutMin=[-200]  OutMax=[200]
  Adjust : Outport
  wires:
  Saturation/1 -> Ki/1
  Memory1/1 -> Sum1/2
  Sum1/1 -> Saturation/1, Memory1/1  "pid_integ"
  Sum6/1 -> Kp/1, dt/1, Memory/1, Sum2/1  "pid_error"
  1/dt/1 -> Kd/1
  Sum2/1 -> 1/dt/1
  dt/1 -> Sum1/1
  Kd/1 -> Sum5/3
  Kp/1 -> Sum5/1
  Sum5/1 -> Adjust/1
  Ki/1 -> Sum5/2
  Memory/1 -> Sum2/2  "pid_prevError"
  Setpoint/1 -> Sum6/1  "pid_desired"
  Measured/1 -> Sum6/2  "measured"

== system ILC_pidQuadsim/Controller/Attitude_controller/PID_Pitch3 ==
  Setpoint : Inport
  Measured : Inport  Port=2
  1/dt : Gain  Gain=250  OutMin=[-200]  OutMax=[200]
  Kd : Gain  Gain=0  OutMin=[-200]  OutMax=[200]
  Ki : Gain  Gain=0  OutMin=[-200]  OutMax=[200]
  Kp : Gain  Gain=3.5  OutMin=[-200]  OutMax=[200]
  Memory : Memory
  Memory1 : Memory
  Saturation : Saturate  UpperLimit=20  LowerLimit=-20
  Sum1 : Sum  Inputs=|++
  Sum2 : Sum  Inputs=|+-
  Sum5 : Sum  Inputs=+++
  Sum6 : Sum  Inputs=+-|
  dt : Gain  Gain=1/250  OutMin=[-200]  OutMax=[200]
  Adjust : Outport
  wires:
  Measured/1 -> Sum6/2  "measured"
  Setpoint/1 -> Sum6/1  "pid_desired"
  Memory/1 -> Sum2/2  "pid_prevError"
  Ki/1 -> Sum5/2
  Sum5/1 -> Adjust/1
  Kp/1 -> Sum5/1
  Kd/1 -> Sum5/3
  dt/1 -> Sum1/1
  Sum2/1 -> 1/dt/1
  1/dt/1 -> Kd/1
  Sum6/1 -> Sum2/1, Memory/1, dt/1, Kp/1  "pid_error"
  Sum1/1 -> Memory1/1, Saturation/1  "pid_integ"
  Memory1/1 -> Sum1/2
  Saturation/1 -> Ki/1

== system ILC_pidQuadsim/Controller/Attitude_controller/PID_Pitch_Rate2 ==
  Setpoint : Inport
  Measured : Inport  Port=2
  Derivative : Derivative
  Integrator Limited : Integrator  LimitOutput=on  UpperSaturationLimit=20  LowerSaturationLimit=-20
  Kd : Gain  Gain=0  OutMin=[-200]  OutMax=[200]
  Ki : Gain  Gain=2  OutMin=[-200]  OutMax=[200]
  Kp : Gain  Gain=3.5  OutMin=[-200]  OutMax=[200]
  Scope : Scope
  Sum5 : Sum  Inputs=+++
  Sum6 : Sum  Inputs=+-|
  Adjust : Outport
  wires:
  Derivative/1 -> Kd/1
  Integrator Limited/1 -> Ki/1, Scope/1
  Sum6/1 -> Kp/1, Integrator Limited/1, Derivative/1  "pid_error"
  Kd/1 -> Sum5/3
  Kp/1 -> Sum5/1
  Sum5/1 -> Adjust/1
  Ki/1 -> Sum5/2
  Setpoint/1 -> Sum6/1  "pid_desired"
  Measured/1 -> Sum6/2  "measured"

== system ILC_pidQuadsim/Controller/Attitude_controller/PID_Roll_Rate1 ==
  Setpoint : Inport
  Measured : Inport  Port=2
  Derivative : Derivative
  Integrator Limited : Integrator  LimitOutput=on  UpperSaturationLimit=20  LowerSaturationLimit=-20
  Kd : Gain  Gain=0  OutMin=[-200]  OutMax=[200]
  Ki : Gain  Gain=2  OutMin=[-200]  OutMax=[200]
  Kp : Gain  Gain=3.5  OutMin=[-200]  OutMax=[200]
  Scope : Scope
  Sum5 : Sum  Inputs=+++
  Sum6 : Sum  Inputs=+-|
  Adjust : Outport
  wires:
  Measured/1 -> Sum6/2  "measured"
  Setpoint/1 -> Sum6/1  "pid_desired"
  Ki/1 -> Sum5/2
  Sum5/1 -> Adjust/1
  Kp/1 -> Sum5/1
  Kd/1 -> Sum5/3
  Sum6/1 -> Derivative/1, Integrator Limited/1, Kp/1  "pid_error"
  Integrator Limited/1 -> Scope/1, Ki/1
  Derivative/1 -> Kd/1

== system ILC_pidQuadsim/Controller/Control_mixer/Configuration_+ ==
  Pitch : Inport
  Roll : Inport  Port=2
  Yaw : Inport  Port=3
  Tau : Inport  Port=4
  Sum{1,9..12} (5 alike) : Sum  Inputs=|++  InputSameDT=on  SaturateOnIntegerOverflow=on  OutDataTypeStr=Inherit: Same as first input
  Sum3 : Sum  Inputs=|--  InputSameDT=on  SaturateOnIntegerOverflow=on  OutDataTypeStr=Inherit: Same as first input
  Sum5 : Sum  Inputs=|-+  InputSameDT=on  SaturateOnIntegerOverflow=on  OutDataTypeStr=Inherit: Same as first input
  Sum7 : Sum  Inputs=|+-  InputSameDT=on  SaturateOnIntegerOverflow=on  OutDataTypeStr=Inherit: Same as first input
  W1 : Outport
  W2 : Outport  Port=2
  W3 : Outport  Port=3
  W4 : Outport  Port=4
  wires:
  Sum5/1 -> Sum11/1
  Yaw/1 -> Sum7/2, Sum5/2, Sum3/2, Sum1/2
  Tau/1 -> Sum11/2, Sum12/2, Sum10/2, Sum9/2
  Sum9/1 -> W1/1
  Pitch/1 -> Sum1/1, Sum5/1
  Roll/1 -> Sum3/1, Sum7/1
  Sum11/1 -> W3/1
  Sum12/1 -> W4/1
  Sum7/1 -> Sum12/1
  Sum10/1 -> W2/1
  Sum1/1 -> Sum9/1
  Sum3/1 -> Sum10/1

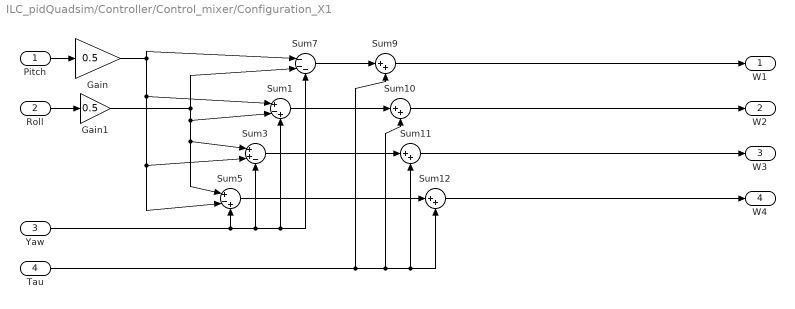
== system ILC_pidQuadsim/Controller/Control_mixer/Configuration_X1 ==
  Pitch : Inport
  Roll : Inport  Port=2
  Yaw : Inport  Port=3
  Tau : Inport  Port=4
  Gain : Gain  Gain=0.5
  Gain1 : Gain  Gain=0.5
  Sum1 : Sum  Inputs=|+-+  InputSameDT=on  SaturateOnIntegerOverflow=on  OutDataTypeStr=Inherit: Same as first input
  Sum{9..12} (4 alike) : Sum  Inputs=|++  InputSameDT=on  SaturateOnIntegerOverflow=on  OutDataTypeStr=Inherit: Same as first input
  Sum3 : Sum  Inputs=|++-  InputSameDT=on  SaturateOnIntegerOverflow=on  OutDataTypeStr=Inherit: Same as first input
  Sum5 : Sum  Inputs=|+-+  InputSameDT=on  SaturateOnIntegerOverflow=on  OutDataTypeStr=Inherit: Same as first input
  Sum7 : Sum  Inputs=|---  InputSameDT=on  SaturateOnIntegerOverflow=on  OutDataTypeStr=Inherit: Same as first input
  W1 : Outport
  W2 : Outport  Port=2
  W3 : Outport  Port=3
  W4 : Outport  Port=4
  wires:
  Sum3/1 -> Sum11/1
  Yaw/1 -> Sum5/3, Sum3/3, Sum7/3, Sum1/3
  Tau/1 -> Sum11/2, Sum12/2, Sum10/2, Sum9/2
  Sum5/1 -> Sum12/1
  Sum7/1 -> Sum9/1
  Sum1/1 -> Sum10/1
  Roll/1 -> Gain1/1
  Pitch/1 -> Gain/1
  Gain/1 -> Sum7/1, Sum1/1, Sum5/2, Sum3/2
  Gain1/1 -> Sum7/2, Sum1/2, Sum5/1, Sum3/1
  Sum9/1 -> W1/1
  Sum10/1 -> W2/1
  Sum11/1 -> W3/1
  Sum12/1 -> W4/1

== system ILC_pidQuadsim/Controller/Position_controller/PID_Roll_Rate2 ==
  Setpoint : Inport
  Measured : Inport  Port=2
  Derivative : Derivative
  Integrator Limited : Integrator  LimitOutput=on  UpperSaturationLimit=0.1  LowerSaturationLimit=-0.1
  Kd : Gain  Gain=0  OutMin=[-200]  OutMax=[200]
  Ki : Gain  Gain=2  OutMin=[-200]  OutMax=[200]
  Kp : Gain  Gain=30  OutMin=[-200]  OutMax=[200]
  Scope : Scope
  Sum5 : Sum  Inputs=+++
  Sum6 : Sum  Inputs=+-|
  Adjust : Outport
  wires:
  Measured/1 -> Sum6/2  "measured"
  Setpoint/1 -> Sum6/1  "pid_desired"
  Ki/1 -> Sum5/2
  Sum5/1 -> Adjust/1
  Kp/1 -> Sum5/1
  Kd/1 -> Sum5/3
  Sum6/1 -> Derivative/1, Integrator Limited/1, Kp/1  "pid_error"
  Integrator Limited/1 -> Scope/1, Ki/1
  Derivative/1 -> Kd/1

== system ILC_pidQuadsim/Controller/Position_controller/PID_Roll_Rate3 ==
  Setpoint : Inport
  Measured : Inport  Port=2
  Derivative : Derivative
  Integrator Limited : Integrator  LimitOutput=on  UpperSaturationLimit=0.1  LowerSaturationLimit=-0.1
  Kd : Gain  Gain=0  OutMin=[-200]  OutMax=[200]
  Ki : Gain  Gain=-2  OutMin=[-200]  OutMax=[200]
  Kp : Gain  Gain=-30  OutMin=[-200]  OutMax=[200]
  Scope : Scope
  Sum5 : Sum  Inputs=+++
  Sum6 : Sum  Inputs=+-|
  Adjust : Outport
  wires:
  Derivative/1 -> Kd/1
  Integrator Limited/1 -> Ki/1, Scope/1
  Sum6/1 -> Kp/1, Integrator Limited/1, Derivative/1  "pid_error"
  Kd/1 -> Sum5/3
  Kp/1 -> Sum5/1
  Sum5/1 -> Adjust/1
  Ki/1 -> Sum5/2
  Setpoint/1 -> Sum6/1  "pid_desired"
  Measured/1 -> Sum6/2  "measured"

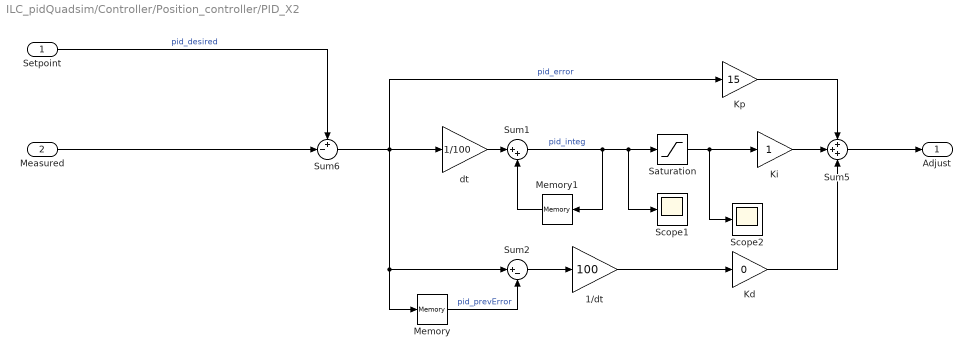
== system ILC_pidQuadsim/Controller/Position_controller/PID_X2 ==
  Setpoint : Inport
  Measured : Inport  Port=2
  1/dt : Gain  Gain=100  OutMin=[-200]  OutMax=[200]
  Kd : Gain  Gain=0  OutMin=[-200]  OutMax=[200]
  Ki : Gain  OutMin=[-200]  OutMax=[200]
  Kp : Gain  Gain=15  OutMin=[-200]  OutMax=[200]
  Memory : Memory
  Memory1 : Memory
  Saturation : Saturate  UpperLimit=0.1  LowerLimit=-0.1
  Scope1 : Scope
  Scope2 : Scope
  Sum1 : Sum  Inputs=|++
  Sum2 : Sum  Inputs=|+-
  Sum5 : Sum  Inputs=+++
  Sum6 : Sum  Inputs=+-|
  dt : Gain  Gain=1/100  OutMin=[-200]  OutMax=[200]
  Adjust : Outport
  wires:
  Measured/1 -> Sum6/2
  Saturation/1 -> Ki/1, Scope2/1
  Memory1/1 -> Sum1/2
  Sum1/1 -> Saturation/1, Scope1/1, Memory1/1  "pid_integ"
  Sum6/1 -> Kp/1, dt/1, Memory/1, Sum2/1  "pid_error"
  1/dt/1 -> Kd/1
  Sum2/1 -> 1/dt/1
  dt/1 -> Sum1/1
  Kd/1 -> Sum5/3
  Kp/1 -> Sum5/1
  Sum5/1 -> Adjust/1
  Ki/1 -> Sum5/2
  Memory/1 -> Sum2/2  "pid_prevError"
  Setpoint/1 -> Sum6/1  "pid_desired"

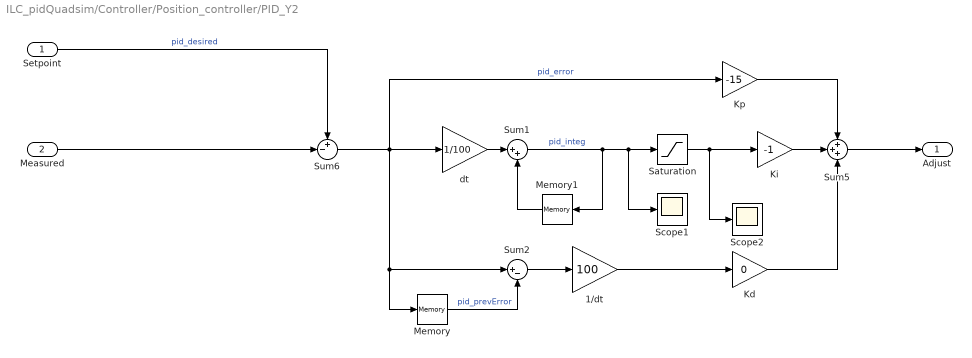
== system ILC_pidQuadsim/Controller/Position_controller/PID_Y2 ==
  Setpoint : Inport
  Measured : Inport  Port=2
  1/dt : Gain  Gain=100  OutMin=[-200]  OutMax=[200]
  Kd : Gain  Gain=0  OutMin=[-200]  OutMax=[200]
  Ki : Gain  Gain=-1  OutMin=[-200]  OutMax=[200]
  Kp : Gain  Gain=-15  OutMin=[-200]  OutMax=[200]
  Memory : Memory
  Memory1 : Memory
  Saturation : Saturate  UpperLimit=0.1  LowerLimit=-0.1
  Scope1 : Scope
  Scope2 : Scope
  Sum1 : Sum  Inputs=|++
  Sum2 : Sum  Inputs=|+-
  Sum5 : Sum  Inputs=+++
  Sum6 : Sum  Inputs=+-|
  dt : Gain  Gain=1/100  OutMin=[-200]  OutMax=[200]
  Adjust : Outport
  wires:
  Measured/1 -> Sum6/2
  Saturation/1 -> Ki/1, Scope2/1
  Memory1/1 -> Sum1/2
  Sum1/1 -> Saturation/1, Scope1/1, Memory1/1  "pid_integ"
  Sum6/1 -> Kp/1, dt/1, Memory/1, Sum2/1  "pid_error"
  1/dt/1 -> Kd/1
  Sum2/1 -> 1/dt/1
  dt/1 -> Sum1/1
  Kd/1 -> Sum5/3
  Kp/1 -> Sum5/1
  Sum5/1 -> Adjust/1
  Ki/1 -> Sum5/2
  Memory/1 -> Sum2/2  "pid_prevError"
  Setpoint/1 -> Sum6/1  "pid_desired"

== system ILC_pidQuadsim/Controller/Rate_controller/PID_Pitch_Rate1 ==
  Setpoint : Inport
  Measured : Inport  Port=2
  1/dt : Gain  Gain=500  OutMin=[-200]  OutMax=[200]
  Kd : Gain  Gain=0  OutMin=[-200]  OutMax=[200]
  Ki : Gain  Gain=0  OutMin=[-200]  OutMax=[200]
  Kp : Gain  Gain=70  OutMin=[-200]  OutMax=[200]
  Memory : Memory
  Memory1 : Memory
  Saturation : Saturate  UpperLimit=33  LowerLimit=-33
  Sum1 : Sum  Inputs=|++
  Sum2 : Sum  Inputs=|+-
  Sum5 : Sum  Inputs=+++
  Sum6 : Sum  Inputs=+-|
  dt : Gain  Gain=1/500  OutMin=[-200]  OutMax=[200]
  Adjust : Outport
  wires:
  Saturation/1 -> Ki/1
  Memory1/1 -> Sum1/2
  Sum1/1 -> Memory1/1, Saturation/1  "pid_integ"
  Sum6/1 -> Kp/1, dt/1, Memory/1, Sum2/1  "pid_error"
  1/dt/1 -> Kd/1
  Sum2/1 -> 1/dt/1
  dt/1 -> Sum1/1
  Kd/1 -> Sum5/3
  Kp/1 -> Sum5/1
  Sum5/1 -> Adjust/1
  Ki/1 -> Sum5/2
  Memory/1 -> Sum2/2  "pid_prevError"
  Setpoint/1 -> Sum6/1  "pid_desired"
  Measured/1 -> Sum6/2  "measured"

== system ILC_pidQuadsim/Controller/Rate_controller/PID_Pitch_Rate3 ==
  Setpoint : Inport
  Measured : Inport  Port=2
  1/dt : Gain  Gain=500  OutMin=[-200]  OutMax=[200]
  Kd : Gain  Gain=0  OutMin=[-200]  OutMax=[200]
  Ki : Gain  Gain=0  OutMin=[-200]  OutMax=[200]
  Kp : Gain  Gain=70  OutMin=[-200]  OutMax=[200]
  Memory : Memory
  Memory1 : Memory
  Saturation : Saturate  UpperLimit=33  LowerLimit=-33
  Sum1 : Sum  Inputs=|++
  Sum2 : Sum  Inputs=|+-
  Sum5 : Sum  Inputs=+++
  Sum6 : Sum  Inputs=+-|
  dt : Gain  Gain=1/500  OutMin=[-200]  OutMax=[200]
  Adjust : Outport
  wires:
  Measured/1 -> Sum6/2  "measured"
  Setpoint/1 -> Sum6/1  "pid_desired"
  Memory/1 -> Sum2/2  "pid_prevError"
  Ki/1 -> Sum5/2
  Sum5/1 -> Adjust/1
  Kp/1 -> Sum5/1
  Kd/1 -> Sum5/3
  dt/1 -> Sum1/1
  Sum2/1 -> 1/dt/1
  1/dt/1 -> Kd/1
  Sum6/1 -> Sum2/1, Memory/1, dt/1, Kp/1  "pid_error"
  Sum1/1 -> Saturation/1, Memory1/1  "pid_integ"
  Memory1/1 -> Sum1/2
  Saturation/1 -> Ki/1

== system ILC_pidQuadsim/Controller/Rate_controller/PID_Roll_Rate1 ==
  Setpoint : Inport
  Measured : Inport  Port=2
  Derivative : Derivative
  Integrator Limited : Integrator  LimitOutput=on  UpperSaturationLimit=1000  LowerSaturationLimit=-1000
  Kd : Gain  Gain=0  OutMin=[-200]  OutMax=[200]
  Ki : Gain  Gain=0  OutMin=[-200]  OutMax=[200]
  Kp : Gain  Gain=70  OutMin=[-200]  OutMax=[200]
  Scope : Scope
  Sum5 : Sum  Inputs=+++
  Sum6 : Sum  Inputs=+-|
  Adjust : Outport
  wires:
  Measured/1 -> Sum6/2  "measured"
  Setpoint/1 -> Sum6/1  "pid_desired"
  Ki/1 -> Sum5/2
  Sum5/1 -> Adjust/1
  Kp/1 -> Sum5/1
  Kd/1 -> Sum5/3
  Sum6/1 -> Derivative/1, Integrator Limited/1, Kp/1  "pid_error"
  Integrator Limited/1 -> Scope/1, Ki/1
  Derivative/1 -> Kd/1

== system ILC_pidQuadsim/Controller/Rate_controller/PID_Roll_Rate3 ==
  Setpoint : Inport
  Measured : Inport  Port=2
  Derivative : Derivative
  Integrator Limited : Integrator  LimitOutput=on  UpperSaturationLimit=1000  LowerSaturationLimit=-1000
  Kd : Gain  Gain=0  OutMin=[-200]  OutMax=[200]
  Ki : Gain  Gain=0  OutMin=[-200]  OutMax=[200]
  Kp : Gain  Gain=70  OutMin=[-200]  OutMax=[200]
  Scope : Scope
  Sum5 : Sum  Inputs=+++
  Sum6 : Sum  Inputs=+-|
  Adjust : Outport
  wires:
  Derivative/1 -> Kd/1
  Integrator Limited/1 -> Ki/1, Scope/1
  Sum6/1 -> Kp/1, Integrator Limited/1, Derivative/1  "pid_error"
  Kd/1 -> Sum5/3
  Kp/1 -> Sum5/1
  Sum5/1 -> Adjust/1
  Ki/1 -> Sum5/2
  Setpoint/1 -> Sum6/1  "pid_desired"
  Measured/1 -> Sum6/2  "measured"

== system ILC_pidQuadsim/Controller2/Altitude_controller/PID_Altitude ==
  Setpoint : Inport
  Measured : Inport  Port=2
  Derivative : Derivative
  Integrator Limited : Integrator  LimitOutput=on  UpperSaturationLimit=1000  LowerSaturationLimit=-1000
  Kd : Gain  Gain=9000  OutMin=[-200]  OutMax=[200]
  Ki : Gain  Gain=3500  OutMin=[-200]  OutMax=[200]
  Kp : Gain  Gain=11000  OutMin=[-200]  OutMax=[200]
  Sum5 : Sum  Inputs=+++
  Sum6 : Sum  Inputs=+-|
  Adjust : Outport
  wires:
  Sum5/1 -> Adjust/1
  Measured/1 -> Sum6/2  "measured"
  Setpoint/1 -> Sum6/1  "pid_desired"
  Ki/1 -> Sum5/2
  Kp/1 -> Sum5/1
  Kd/1 -> Sum5/3
  Sum6/1 -> Derivative/1, Integrator Limited/1, Kp/1  "pid_error"
  Integrator Limited/1 -> Ki/1
  Derivative/1 -> Kd/1

== system ILC_pidQuadsim/Controller2/Attitude_controller/PID_Pitch1 ==
  Setpoint : Inport
  Measured : Inport  Port=2
  1/dt : Gain  Gain=250  OutMin=[-200]  OutMax=[200]
  Kd : Gain  Gain=0  OutMin=[-200]  OutMax=[200]
  Ki : Gain  Gain=0  OutMin=[-200]  OutMax=[200]
  Kp : Gain  Gain=3.5  OutMin=[-200]  OutMax=[200]
  Memory : Memory
  Memory1 : Memory
  Saturation : Saturate  UpperLimit=20  LowerLimit=-20
  Sum1 : Sum  Inputs=|++
  Sum2 : Sum  Inputs=|+-
  Sum5 : Sum  Inputs=+++
  Sum6 : Sum  Inputs=+-|
  dt : Gain  Gain=1/250  OutMin=[-200]  OutMax=[200]
  Adjust : Outport
  wires:
  Measured/1 -> Sum6/2  "measured"
  Setpoint/1 -> Sum6/1  "pid_desired"
  Memory/1 -> Sum2/2  "pid_prevError"
  Ki/1 -> Sum5/2
  Sum5/1 -> Adjust/1
  Kp/1 -> Sum5/1
  Kd/1 -> Sum5/3
  dt/1 -> Sum1/1
  Sum2/1 -> 1/dt/1
  1/dt/1 -> Kd/1
  Sum6/1 -> Sum2/1, Memory/1, dt/1, Kp/1  "pid_error"
  Sum1/1 -> Memory1/1, Saturation/1  "pid_integ"
  Memory1/1 -> Sum1/2
  Saturation/1 -> Ki/1

== system ILC_pidQuadsim/Controller2/Attitude_controller/PID_Pitch3 ==
  Setpoint : Inport
  Measured : Inport  Port=2
  1/dt : Gain  Gain=250  OutMin=[-200]  OutMax=[200]
  Kd : Gain  Gain=0  OutMin=[-200]  OutMax=[200]
  Ki : Gain  Gain=0  OutMin=[-200]  OutMax=[200]
  Kp : Gain  Gain=3.5  OutMin=[-200]  OutMax=[200]
  Memory : Memory
  Memory1 : Memory
  Saturation : Saturate  UpperLimit=20  LowerLimit=-20
  Sum1 : Sum  Inputs=|++
  Sum2 : Sum  Inputs=|+-
  Sum5 : Sum  Inputs=+++
  Sum6 : Sum  Inputs=+-|
  dt : Gain  Gain=1/250  OutMin=[-200]  OutMax=[200]
  Adjust : Outport
  wires:
  Saturation/1 -> Ki/1
  Memory1/1 -> Sum1/2
  Sum1/1 -> Saturation/1, Memory1/1  "pid_integ"
  Sum6/1 -> Kp/1, dt/1, Memory/1, Sum2/1  "pid_error"
  1/dt/1 -> Kd/1
  Sum2/1 -> 1/dt/1
  dt/1 -> Sum1/1
  Kd/1 -> Sum5/3
  Kp/1 -> Sum5/1
  Sum5/1 -> Adjust/1
  Ki/1 -> Sum5/2
  Memory/1 -> Sum2/2  "pid_prevError"
  Setpoint/1 -> Sum6/1  "pid_desired"
  Measured/1 -> Sum6/2  "measured"
